simulink model "friction_model_stiction_coloumb"  (R2016a)
settings: Solver=VariableStepAuto  StartTime=0.0  StopTime=10.0  RelTol=1e-3
undefined symbols (not defined in the file): g, gammaC, gammaX, gammaY, h, l, lcm, ld, m, r, w
settings Model: Creator=mgreiff  LastModifiedBy=mgreiff

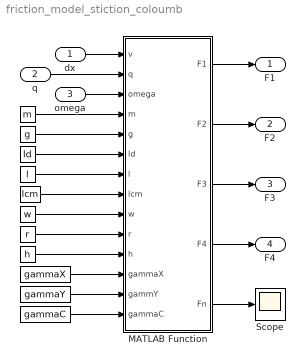
== system friction_model_stiction_coloumb ==
  dx : Inport  PortDimensions=3
  q : Inport  Port=2  PortDimensions=4
  omega : Inport  Port=3  PortDimensions=3
  " " : Constant  Value=ld
  "  " : Constant  Value=m
  "   " : Constant  Value=gammaX
  "    " : Constant  Value=gammaY
  "     " : Constant  Value=gammaC
  "      " : Constant  Value=w
  "       " : Constant  Value=r
  "        " : Constant  Value=h
  "          " : Constant  Value=g
  "              " : Constant  Value=l
  "               " : Constant  Value=lcm
  MATLAB Function : MATLAB Function  TreatAsAtomicUnit=on
  Scope : Scope
  F1 : Outport  PortDimensions=3
  F2 : Outport  Port=2  PortDimensions=3
  F3 : Outport  Port=3  PortDimensions=3
  F4 : Outport  Port=4  PortDimensions=3
  wires:
  dx/1 -> MATLAB Function/1(v)
  MATLAB Function/4(F4) -> F4/1
  MATLAB Function/3(F3) -> F3/1
  MATLAB Function/2(F2) -> F2/1
  MATLAB Function/1(F1) -> F1/1
  omega/1 -> MATLAB Function/3(omega)
  q/1 -> MATLAB Function/2(q)
  "  "/1 -> MATLAB Function/4(m)
  "          "/1 -> MATLAB Function/5(g)
  " "/1 -> MATLAB Function/6(ld)
  "              "/1 -> MATLAB Function/7(l)
  "               "/1 -> MATLAB Function/8(lcm)
  "      "/1 -> MATLAB Function/9(w)
  "       "/1 -> MATLAB Function/10(r)
  "        "/1 -> MATLAB Function/11(h)
  "   "/1 -> MATLAB Function/12(gammaX)
  "    "/1 -> MATLAB Function/13(gammY)
  "     "/1 -> MATLAB Function/14(gammaC)
  MATLAB Function/5(Fn) -> Scope/1

== matlab function friction_model_stiction_coloumb/MATLAB Function ==
  data: v input; q input; omega input; m input; g input; ld input; l input; lcm input; w input; r input; h input; F1 output; F2 output; F3 output; F4 output; gammaX input; gammY input; gammaC input; Fn output
function [F1, F2, F3, F4, Fn] = fcn(v, q, omega, m, g, ld, l, lcm, w, r, h, gammaX, gammY, gammaC)
%#codegen
d1 = [0,-w,0]';
d2 = [0,w,0]';
d3 = [l,w,0]';
d4 = [l,-w,0]';
omega = [0;0;0];
F1 = -gammaC.*(cross(d1, omega) + v);
F2 = -gammaC.*(cross(d2, omega) + v);
F3 = -gammaC.*(cross(d3, omega) + v);
F4 = -gammaC.*(cross(d4, omega) + v);
F1(3) = 0;
F2(3) = 0;
F3(3) = 0;
F4(3) = 0;
Fn = [norm(F1), norm(F2), norm(F3), norm(F4)]; % Norms of the fiction forces for debugging
end
